simulink model "simulation"  (R2023b)
settings: Solver=VariableStepAuto  StartTime=0.0  StopTime=10.0  RelTol=1e-3
values from neighbouring files (symbols this model uses):
  A1 = 2    [script.m]
  a1 = (AW1 * sqrt(2 * g * H1)) / H1    [script.m]
  A2 = 8    [script.m]
  a2 = (AW2 * sqrt(2 * g * H2)) / H2    [script.m]
  flow_input_step_1 = 0    [script.m]
  flow_input_step_2 = 0.1 * flow_input_max_2    [script.m]
  initial_flow_input_1 = flow_inputs_vec_1(i)    [script.m]
  initial_flow_input_2 = flow_input_max_2    [script.m]
  initial_height_1 = flow_input_max_1 / a1    [script.m]
  initial_height_2 = (flow_inputs_vec_2(i) + flow_input_max_1) / a2    [script.m]
  T0 = 2    [script.m]
settings Model: Creator=igorkrzywda  LastModifiedBy=igorkrzywda

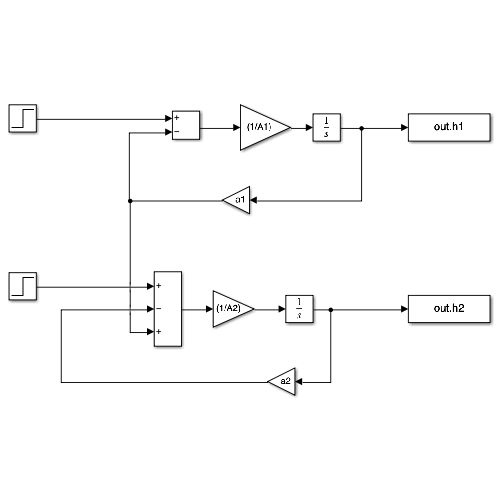
[thumbnail: Simulink's stored preview of the top-level diagram]
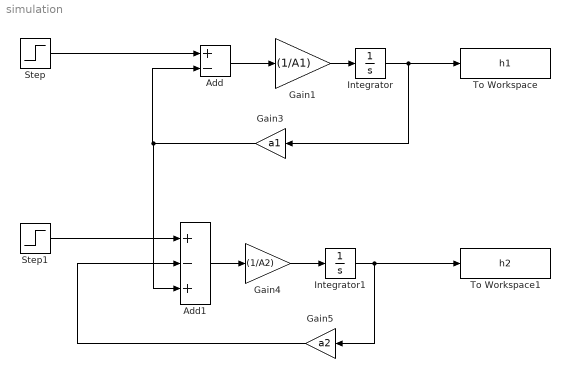
== system simulation ==
  Add : Sum  Inputs=+-
  Add1 : Sum  Inputs=+-+
  Gain1 : Gain  Gain=(1/A1)
  Gain3 : Gain  Gain=a1
  Gain4 : Gain  Gain=(1/A2)
  Gain5 : Gain  Gain=a2
  Integrator : Integrator  InitialCondition=initial_height_1
  Integrator1 : Integrator  InitialCondition=initial_height_2
  Step : Step  Time=T0  Before=initial_flow_input_1  After=initial_flow_input_1 + flow_input_step_1  SampleTime=0
  Step1 : Step  Time=T0  Before=initial_flow_input_2  After=initial_flow_input_2 + flow_input_step_2  SampleTime=0
  To Workspace : ToWorkspace  VariableName=h1  SampleTime=-1
  To Workspace1 : ToWorkspace  VariableName=h2  SampleTime=-1
  wires:
  Integrator/1 -> To Workspace/1, Gain3/1
  Integrator1/1 -> To Workspace1/1, Gain5/1
  Add/1 -> Gain1/1
  Gain1/1 -> Integrator/1
  Gain3/1 -> Add1/3, Add/2
  Add1/1 -> Gain4/1
  Gain4/1 -> Integrator1/1
  Gain5/1 -> Add1/2
  Step/1 -> Add/1
  Step1/1 -> Add1/1
